simulink model "Lab_1"  (R2021b)
settings: Solver=VariableStepAuto  StartTime=0.0  StopTime=10.0  RelTol=1e-3
settings Model: Creator=Ivershin  LastModifiedBy=Ivershin

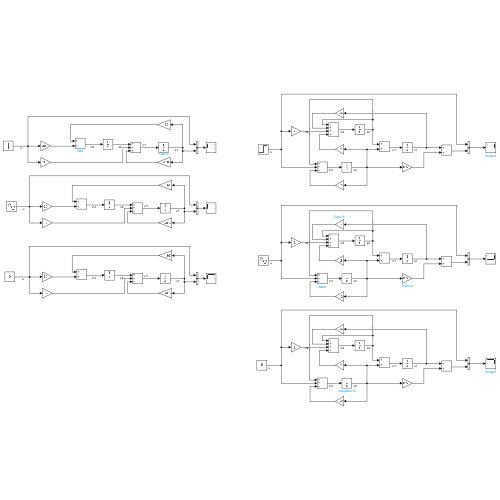
[thumbnail: Simulink's stored preview of the top-level diagram]
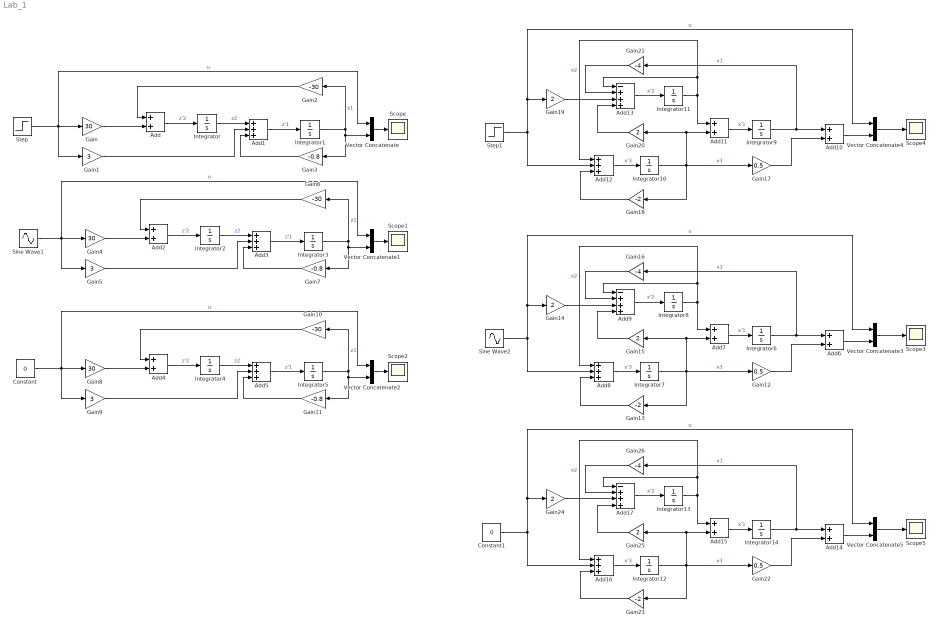
== system Lab_1 ==
  Add{,2,4,6..7,10..11,14..15} (9 alike) : Sum
  Add{1,3,5,8,12,16} (6 alike) : Sum  Inputs=+++
  Add13 : Sum  Inputs=-+++
  Add17 : Sum  Inputs=-+++
  Add9 : Sum  Inputs=-+++
  Constant : Constant  Value=0
  Constant1 : Constant  Value=0
  Gain : Gain  Gain=30
  Gain1 : Gain  Gain=3
  Gain10 : Gain  Gain=-30
  Gain11 : Gain  Gain=-0.8
  Gain12 : Gain  Gain=0.5
  Gain13 : Gain  Gain=-2
  Gain{14..15,19..20,24..25} (6 alike) : Gain  Gain=2
  Gain16 : Gain  Gain=-4
  Gain17 : Gain  Gain=0.5
  Gain18 : Gain  Gain=-2
  Gain2 : Gain  Gain=-30
  Gain21 : Gain  Gain=-4
  Gain22 : Gain  Gain=0.5
  Gain23 : Gain  Gain=-2
  Gain26 : Gain  Gain=-4
  Gain3 : Gain  Gain=-0.8
  Gain4 : Gain  Gain=30
  Gain5 : Gain  Gain=3
  Gain6 : Gain  Gain=-30
  Gain7 : Gain  Gain=-0.8
  Gain8 : Gain  Gain=30
  Gain9 : Gain  Gain=3
  Integrator{,1..3,6..12} (11 alike) : Integrator
  Integrator13 : Integrator  InitialCondition=-2
  Integrator14 : Integrator  InitialCondition=0.5
  Integrator4 : Integrator  InitialCondition=1
  Integrator5 : Integrator  InitialCondition=1.3
  Scope{,1..5} (6 alike) : Scope
  Sine Wave1 : Sin  Amplitude=2  SampleTime=0
  Sine Wave2 : Sin  Amplitude=2  SampleTime=0
  Step : Step  SampleTime=0
  Step1 : Step  SampleTime=0
  Vector Concatenate{,1..5} (6 alike) : Concatenate
  wires:
  Step/1 -> Vector Concatenate/1, Gain1/1, Gain/1  "u"
  Gain/1 -> Add/2
  Add/1 -> Integrator/1  "z'2"
  Integrator/1 -> Add1/1  "z2"
  Add1/1 -> Integrator1/1  "z'1"
  Integrator1/1 -> Vector Concatenate/2, Gain3/1, Gain2/1  "z1"
  Gain1/1 -> Add1/2
  Gain2/1 -> Add/1
  Gain3/1 -> Add1/3
  Integrator3/1 -> Vector Concatenate1/2, Gain7/1, Gain6/1  "z1"
  Add3/1 -> Integrator3/1  "z'1"
  Sine Wave1/1 -> Vector Concatenate1/1, Gain5/1, Gain4/1  "u"
  Gain6/1 -> Add2/1
  Gain5/1 -> Add3/2
  Gain7/1 -> Add3/3
  Integrator2/1 -> Add3/1  "z2"
  Gain4/1 -> Add2/2
  Add2/1 -> Integrator2/1  "z'2"
  Vector Concatenate/1 -> Scope/1
  Vector Concatenate1/1 -> Scope1/1
  Vector Concatenate2/1 -> Scope2/1
  Add4/1 -> Integrator4/1  "z'2"
  Integrator4/1 -> Add5/1  "z2"
  Constant/1 -> Vector Concatenate2/1, Gain9/1, Gain8/1  "u"
  Gain11/1 -> Add5/3
  Gain9/1 -> Add5/2
  Gain8/1 -> Add4/2
  Gain10/1 -> Add4/1
  Add5/1 -> Integrator5/1  "z'1"
  Integrator5/1 -> Vector Concatenate2/2, Gain11/1, Gain10/1  "z1"
  Vector Concatenate3/1 -> Scope3/1
  Add6/1 -> Vector Concatenate3/2
  Integrator6/1 -> Gain16/1, Add6/1  "x1"
  Gain12/1 -> Add6/2
  Integrator7/1 -> Gain15/1, Add7/2, Gain12/1, Gain13/1  "x3"
  Add7/1 -> Integrator6/1  "x'1"
  Add8/1 -> Integrator7/1  "x'3"
  Sine Wave2/1 -> Gain14/1, Vector Concatenate3/1, Add8/2  "u"
  Gain13/1 -> Add8/3
  Gain14/1 -> Add9/3
  Gain15/1 -> Add9/4
  Gain16/1 -> Add9/2
  Add9/1 -> Integrator8/1  "x'2"
  Integrator8/1 -> Add7/1, Add8/1, Add9/1  "x2"
  Step1/1 -> Gain19/1, Vector Concatenate4/1, Add12/2  "u"
  Gain21/1 -> Add13/2
  Gain19/1 -> Add13/3
  Integrator9/1 -> Gain21/1, Add10/1  "x1"
  Gain20/1 -> Add13/4
  Integrator11/1 -> Add11/1, Add12/1, Add13/1  "x2"
  Gain18/1 -> Add12/3
  Integrator10/1 -> Gain20/1, Add11/2, Gain17/1, Gain18/1  "x3"
  Add10/1 -> Vector Concatenate4/2
  Add12/1 -> Integrator10/1  "x'3"
  Add13/1 -> Integrator11/1  "x'2"
  Gain17/1 -> Add10/2
  Add11/1 -> Integrator9/1  "x'1"
  Vector Concatenate4/1 -> Scope4/1
  Constant1/1 -> Gain24/1, Vector Concatenate5/1, Add16/2  "u"
  Add15/1 -> Integrator14/1  "x'1"
  Gain22/1 -> Add14/2
  Add17/1 -> Integrator13/1  "x'2"
  Add16/1 -> Integrator12/1  "x'3"
  Add14/1 -> Vector Concatenate5/2
  Integrator12/1 -> Gain25/1, Add15/2, Gain22/1, Gain23/1  "x3"
  Vector Concatenate5/1 -> Scope5/1
  Integrator13/1 -> Add15/1, Add16/1, Add17/1  "x2"
  Gain23/1 -> Add16/3
  Gain25/1 -> Add17/4
  Integrator14/1 -> Gain26/1, Add14/1  "x1"
  Gain26/1 -> Add17/2
  Gain24/1 -> Add17/3
